simulink model "V2X_UDP_SCLX_Control_2019b"  (R2019b)
settings: Solver=FixedStepDiscrete  StartTime=0.0  StopTime=Inf  FixedStep=0.01  RelTol=1e-3
PostLoadFcn:
  | if any(exist('dsrtsu_mdlpostloadfcn', 'file') ~= 0), dsrtsu_mdlpostloadfcn('Execute', bdroot); end
InitFcn:
  | , if any(exist('rtifpga_mdlclblib', 'file') ~= 0), rtifpga_mdlclblib('Init', bdroot); end,
  | , if any(exist('dsmpb_private', 'file') ~= 0), dsmpb_private('dsmpb_mdlclblib', 'Init', bdroot); end,
values from neighbouring files (symbols this model uses):
  CtrlZone_Length = 250    [HDVPSG_DelayComp_NewRef_RealDrop_script_case1.m]
  High_TRFC = 1    [HDVPSG_DelayComp_NewRef_RealDrop_script_case1.m]
  PSG_AMAX = 3.2    [HDVPSG_DelayComp_NewRef_RealDrop_script_case1.m]
  PSG_AMIN = -6    [HDVPSG_DelayComp_NewRef_RealDrop_script_case1.m]
  PSG_first_v0 = 13    [HDVPSG_DelayComp_NewRef_RealDrop_script_case1.m]
  PSG_HighMu_D = 15    [HDVPSG_DelayComp_NewRef_RealDrop_script_case1.m]
  PSG_HighMu_I = 125    [HDVPSG_DelayComp_NewRef_RealDrop_script_case1.m]
  PSG_HighMu_P = 75    [HDVPSG_DelayComp_NewRef_RealDrop_script_case1.m]
  PSG_HighMu_TRFC = 0.8    [HDVPSG_DelayComp_NewRef_RealDrop_script_case1.m]
  PSG_LowMu_D = 12    [HDVPSG_DelayComp_NewRef_RealDrop_script_case1.m]
  PSG_LowMu_I = 64    [HDVPSG_DelayComp_NewRef_RealDrop_script_case1.m]
  PSG_LowMu_P = 48    [HDVPSG_DelayComp_NewRef_RealDrop_script_case1.m]
  PSG_LowMu_TRFC = 0.7    [HDVPSG_DelayComp_NewRef_RealDrop_script_case1.m]
  Q_Leader = 1    [HDVPSG_DelayComp_NewRef_RealDrop_script_case1.m]
  R_Leader = 20    [HDVPSG_DelayComp_NewRef_RealDrop_script_case1.m]
  T_ADE = 0.01    [HDVPSG_DelayComp_NewRef_RealDrop_script_case1.m]
  V_MAX = 40    [HDVPSG_DelayComp_NewRef_RealDrop_script_case1.m]
  V_MIN = 0    [HDVPSG_DelayComp_NewRef_RealDrop_script_case1.m]
undefined symbols (not defined in the file or in its folder): BETA_PSG_Leader, DiscIntNeverNeededParam, UT
libraries: simulink x4, dsmpblib x3
(part 1 of 3)
PreSaveFcn:
  | , if any(exist('dsmpb_private', 'file') ~= 0), dsmpb_private('dsmpb_mdlclblib', 'PreSave', bdroot); end,
CloseFcn:
  | , if any(exist('dsmpb_private', 'file') ~= 0), dsmpb_private('dsmpb_mdlclblib', 'Close', bdroot); end,
settings Model: DSRTSU_INTERNAL_RTIFPGA=200  DSRTSU_INTERNAL_RTISTBM_VER=22.2  DSMPB_ID_DATA={'1507',struct('BlockId','4137d8dd-4dad-4738-91c2-dd6ff22676c4','SignalIds',{{'2f3c0435-b5e6-43b5-a9a2-000eb5ecd229','997bbe15-e0e0-497e-95bc-98f0fbf39b57','0a3da5c5-423a-4b8d-b8d6-f3d0dcb59be2','87608d43-6927-4eb2-b378-ef61d2c19c9c','31e7d2b2-d685-4e77-a494-9395bd212b5d'}}),'1508',struct('BlockId','126ee60d-7173-4c59-ba7e-271ea2a4b692','SignalIds',{{'920c37f5-62e2-421b-87a3-b94423156c86','a9e93576-ca34-4bf6-b67a-2aec0185b5c4'}}),'1509',struct('BlockId','8da95892-a18c-4093-97c9-87f44c323683','SignalIds',{{'7a534e5d-6e34-444f-b618-91e9534136ef'}})}  Creator=znq  LastModifiedBy=Administrator
settings OptimizationCC: BlockReduction=off  ConditionallyExecuteInputs=off  OptimizeBlockIOStorage=off  BufferReuse=off
settings DebuggingCC: TasksWithSamePriorityMsg=none  UnconnectedInputMsg=none  UnconnectedOutputMsg=none  UnconnectedLineMsg=none  SFMachineParentedDataDiag=error
settings HardwareCC: ProdBitPerLong=64  ProdLargestAtomicInteger=Integer  ProdWordSize=32  ProdLongLongMode=on  ProdHWDeviceType=Custom Processor->Custom
settings ModelReferenceCC: EnableParallelModelReferenceBuilds=on
settings RTWCC: Description=dSPACE Target DSRT - Generates SIC files for import by ConfigurationDesk and VEOS. Provides code generation for Simulink models imported in ConfigurationDesk.  SystemTargetFile=dsrt.tlc  GenCodeOnly=on  MakeCommand=make_dsrt  TemplateMakefile=dsrt_default_tmf  RTWVerbose=off  TargetLang=C++
settings CodeAppCC: MaxIdLength=95
settings STFCustomTargetCC: TargetLangStandard=C++03 (ISO)  ParMdlRefBuildCompliant=on  SystemTargetFile=dsrt.tlc
settings GRTTargetCC: TargetLangStandard=C++03 (ISO)  CompOptLevelCompliant=off  ConcurrentExecutionCompliant=off  CombineOutputUpdateFcns=off  MatFileLogging=off  CPPClassGenCompliant=off  UseToolchainInfoCompliant=off

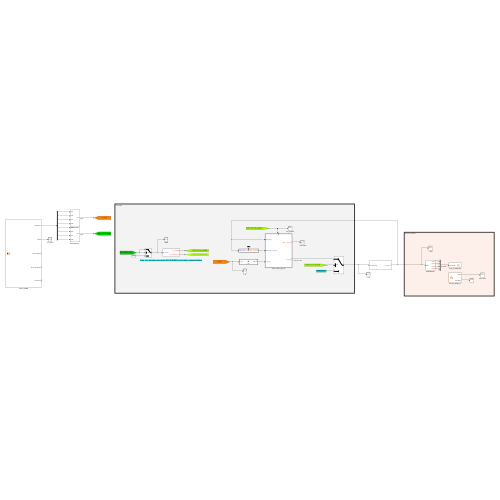
[thumbnail: Simulink's stored preview of the top-level diagram]
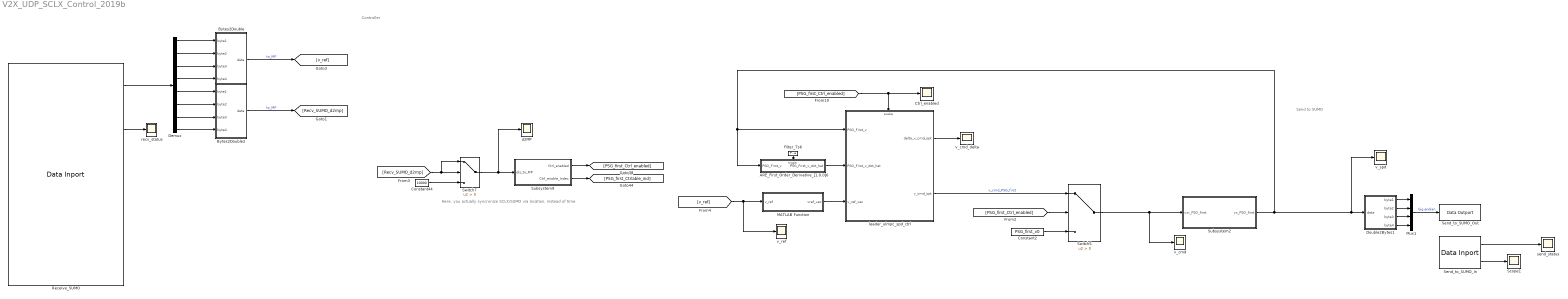
== system V2X_UDP_SCLX_Control_2019b ==
  note: Here, you actually syncronize SCLX/SUMO via location, instead of time
  note: Controller
  note: Send to SUMO
  ARE_First_Order_Derivative_[1,0,0]6 : Subsystem  TreatAsAtomicUnit=on
  Bytes2Double : Subsystem
  Bytes2Double2 : Subsystem
  Constant2 : Constant  Value=PSG_first_v0
  Constant44 : Constant  Value=10000
  Ctrl_enabled : Scope
  Demux : Demux  Outputs=8
  Double2Bytes1 : Subsystem
  Filter_Ts6 : DiscretePulseGenerator  PulseType=Time based  Period=T_ADE*2  PulseWidth=50
  MATLAB Function : MATLAB Function  TreatAsAtomicUnit=on
  Mux1 : Mux
  Receive_SUMO : dsmpblib/Data Inport  Priority=10000
      settings: SourceProductName=dSPACE Model Interface Package for Simulink (MIPS)
  Scope1 : Scope
  Send_to_SUMO_In : dsmpblib/Data Inport  Priority=10000
      settings: SourceProductName=dSPACE Model Interface Package for Simulink (MIPS)
  Send_to_SUMO_Out : dsmpblib/Data Outport  Priority=-10000
      settings: SourceProductName=dSPACE Model Interface Package for Simulink (MIPS)
  Subsystem2 : Subsystem
  Subsystem9 : Subsystem
  Switch5 : Switch  Criteria=u2 > Threshold
  Switch7 : Switch  Criteria=u2 > Threshold
  d2MP : Scope
  leader_ulmpc_spd_ctrl : Subsystem
  recv_status : Scope
  send_status : Scope
  v_cmd : Scope
  v_cmd_delta : Scope
  v_ref : Scope
  v_spd : Scope
  wires:
  Double2Bytes1/4(byte4) -> Mux1/4
  Double2Bytes1/3(byte3) -> Mux1/3
  Double2Bytes1/2(byte2) -> Mux1/2
  Double2Bytes1/1(byte1) -> Mux1/1
  Filter_Ts6/1 -> ARE_First_Order_Derivative_[1,0,0]6/Trigger
  Subsystem9/2(Ctrl_enable_Index) -> [PSG_first_Ctrlable_ind]
  Switch7/1 -> d2MP/1, Subsystem9/1(dis_to_MP)
  Constant44/1 -> Switch7/3
  [PSG_first_Ctrl_enabled] -> leader_ulmpc_spd_ctrl/Enable, Ctrl_enabled/1
  leader_ulmpc_spd_ctrl/2(v_cmd_opt) -> Switch5/1  "v_cmd_PSG_first"
  Subsystem9/1(Ctrl_enabled) -> [PSG_first_Ctrl_enabled]
  ARE_First_Order_Derivative_[1,0,0]6/1(PSG_First_v_dot_hat) -> leader_ulmpc_spd_ctrl/2(PSG_First_v_dot_hat)
  Constant2/1 -> Switch5/3
  [PSG_first_Ctrl_enabled] -> Switch5/2
  Switch5/1 -> v_cmd/1, Subsystem2/1(vxr_PSG_first)
  Mux1/1 -> Send_to_SUMO_Out/1  "big endian"
  leader_ulmpc_spd_ctrl/1(delta_v_cmd_opt) -> v_cmd_delta/1
  Subsystem2/1(vx_PSG_first) -> ARE_First_Order_Derivative_[1,0,0]6/1(PSG_First_v), leader_ulmpc_spd_ctrl/1(PSG_First_v), v_spd/1, Double2Bytes1/1(data)
  MATLAB Function/1(vref_vec) -> leader_ulmpc_spd_ctrl/3(v_ref_vec)
  [v_ref] -> v_ref/1, MATLAB Function/1(v_ref)
  Send_to_SUMO_In/1 -> send_status/1
  Send_to_SUMO_In/2 -> Scope1/1
  Receive_SUMO/1 -> Demux/1
  Receive_SUMO/2 -> recv_status/1
  Demux/1 -> Bytes2Double/1(byte1)
  Demux/2 -> Bytes2Double/2(byte2)
  Demux/3 -> Bytes2Double/3(byte3)
  Demux/4 -> Bytes2Double/4(byte4)
  Demux/5 -> Bytes2Double2/1(byte1)
  Demux/6 -> Bytes2Double2/2(byte2)
  Demux/7 -> Bytes2Double2/3(byte3)
  Demux/8 -> Bytes2Double2/4(byte4)
  Bytes2Double/1(data) -> [v_ref]  "to_MP"
  Bytes2Double2/1(data) -> [Recv_SUMO_d2mp]  "to_MP"
  [Recv_SUMO_d2mp] -> Switch7/1, Switch7/2

== system V2X_UDP_SCLX_Control_2019b/ARE_First_Order_Derivative_[1,0,0]6 ==
  PSG_First_v : Inport
  Trigger : TriggerPort  TriggerType=either  VariantControl=Variant  ZeroCross=off  PortDimensions=1
  Constant : Constant  Value=T_ADE
  Constant1 : Constant  Value=PSG_first_v0
  MATLAB Function : MATLAB Function  TreatAsAtomicUnit=on
  PSG_First_v_dot_hat : Outport  VectorParamsAs1DForOutWhenUnconnected=off
  wires:
  Constant1/1 -> MATLAB Function/3(u_init)
  PSG_First_v/1 -> MATLAB Function/1(U)
  MATLAB Function/1(Dot_U) -> PSG_First_v_dot_hat/1
  Constant/1 -> MATLAB Function/2(Ts)

== system V2X_UDP_SCLX_Control_2019b/Bytes2Double ==
  byte1 : Inport
  byte2 : Inport  Port=2
  byte3 : Inport  Port=3
  byte4 : Inport  Port=4
  Data Type Conversion2 : DataTypeConversion
  MATLAB Function2 : MATLAB Function  TreatAsAtomicUnit=on
  data : Outport
  wires:
  byte1/1 -> MATLAB Function2/1(byte1)
  byte3/1 -> MATLAB Function2/3(byte3)
  MATLAB Function2/1(float32) -> Data Type Conversion2/1
  byte4/1 -> MATLAB Function2/4(byte4)
  Data Type Conversion2/1 -> data/1
  byte2/1 -> MATLAB Function2/2(byte2)

== system V2X_UDP_SCLX_Control_2019b/Bytes2Double2 ==
  byte1 : Inport
  byte2 : Inport  Port=2
  byte3 : Inport  Port=3
  byte4 : Inport  Port=4
  Data Type Conversion2 : DataTypeConversion
  MATLAB Function2 : MATLAB Function  TreatAsAtomicUnit=on
  data : Outport
  wires:
  byte2/1 -> MATLAB Function2/2(byte2)
  Data Type Conversion2/1 -> data/1
  byte4/1 -> MATLAB Function2/4(byte4)
  MATLAB Function2/1(float32) -> Data Type Conversion2/1
  byte3/1 -> MATLAB Function2/3(byte3)
  byte1/1 -> MATLAB Function2/1(byte1)

== system V2X_UDP_SCLX_Control_2019b/Double2Bytes1 ==
  data : Inport
  MATLAB Function3 : MATLAB Function  TreatAsAtomicUnit=on
  Saturation : Saturate  UpperLimit=1e6  LowerLimit=-1e6
  byte1 : Outport
  byte2 : Outport  Port=2
  byte3 : Outport  Port=3
  byte4 : Outport  Port=4
  wires:
  Saturation/1 -> MATLAB Function3/1(defloatMe)
  MATLAB Function3/4(byte4) -> byte4/1
  MATLAB Function3/1(byte1) -> byte1/1
  MATLAB Function3/2(byte2) -> byte2/1
  data/1 -> Saturation/1
  MATLAB Function3/3(byte3) -> byte3/1

== system V2X_UDP_SCLX_Control_2019b/Subsystem2 ==
  vxr_PSG_first : Inport
  Constant56 : Constant  Value=PSG_first_v0
  PSG_first : Subsystem
  Subsystem4 : Subsystem
  Subsystem5 : Subsystem
  Subsystem6 : Subsystem
  Subsystem7 : Subsystem
  Terminator : Terminator
  vx_PSG_first : Outport
  wires:
  vxr_PSG_first/1 -> PSG_first/1(vxr)
  Constant56/1 -> PSG_first/6(v_ini)
  Subsystem4/1(PSG_P) -> PSG_first/2(PID_P)
  Subsystem5/1(PSG_I) -> PSG_first/3(PID_I)
  Subsystem6/1(PSG_D) -> PSG_first/4(PID_D)
  Subsystem7/1(PSG_Mu) -> PSG_first/5(TRFC)
  PSG_first/1(vx) -> vx_PSG_first/1
  PSG_first/2(ax_) -> Terminator/1

== system V2X_UDP_SCLX_Control_2019b/Subsystem9 ==
  dis_to_MP : Inport
  Add5 : Sum
  Compare To Constant1 : simulink/Logic and Bit Operations/Compare To Constant  relop=<=  const=CtrlZone_Length  OutDataTypeStr=boolean
  Compare To Constant2 : simulink/Logic and Bit Operations/Compare To Constant  relop=>  const=0  OutDataTypeStr=boolean
  Data Type Conversion : DataTypeConversion
  Delay : Delay  DelayLength=1
  Ctrl_enabled : Outport
  Ctrl_enable_Index : Outport  Port=2
  wires:
  Data Type Conversion/1 -> Add5/1
  Delay/1 -> Ctrl_enable_Index/1, Add5/2, Compare To Constant2/1
  Add5/1 -> Delay/1
  Compare To Constant2/1 -> Ctrl_enabled/1
  Compare To Constant1/1 -> Data Type Conversion/1
  dis_to_MP/1 -> Compare To Constant1/1

== system V2X_UDP_SCLX_Control_2019b/leader_ulmpc_spd_ctrl ==
  note: CVXGEN only support C compiler. So, this is another reason why you cannot build CVXGEN and SUMO (C++11) code together into SCLX
  note: After test the CVXGEN in a complete Simulink model, you need to separate the CVXGEN file into a Ctrl.slx file to be built into SCLX.
      |
      | Please first delete the generated CVXGEN file from the last local compilation.
      | After you analyze the Ctrl.slx, you will find the CVXGEN related wrapper, etc will automatically appear. Then, make sure the Code Gen setup in Simulink is set to C, instead of C++. Then, you can let CfgDesk to build.
  PSG_First_v : Inport
  PSG_First_v_dot_hat : Inport  Port=2
  v_ref_vec : Inport  Port=3
  Enable : EnablePort
  Constant42 : Constant  Value=Q_Leader
  Constant43 : Constant  Value=R_Leader
  Constant54 : Constant  Value=PSG_AMAX*T_ADE
  Constant55 : Constant  Value=PSG_AMIN*T_ADE
  Constant57 : Constant  Value=V_MAX
  Constant58 : Constant  Value=V_MIN
  Constant59 : Constant  Value=T_ADE
  Constant61 : Constant  Value=BETA_PSG_Leader
  Memory2 : Memory  InitialCondition=PSG_first_v0
  Rate Transition{6,48..50,68,70..80} (16 alike) : RateTransition
  S-Function Builder : S-Function  FunctionName=ULMPC_Spd_Ctrl  SFunctionModules=ULMPC_Spd_Ctrl_wrapper solver util matrix_support ldl  SFunctionDeploymentMode=off  EnableBusSupport=off  mask(S-Function Builder){}
      mask help: Simulink:masks:SFunctionBuilder_MD
      mask init:
      | val = [[.9  0.75 0.75 1 1 .9 .9 1]',[1 1 0.75 0.75 .9 .9 1 .9]'];try , sys = get_param(gcb,'SfunBuilderFcnName');if isempty(sys), sys = get_param(gcb,'FunctionName'); end,catch, sys = get_param(gcb,'FunctionName'); end
      settings: CopyFcn=set_param(gcbh,'LinkStatus','none')  OpenFcn=sfunctionwizard(gcbh)
      mask Display:
      | plot(val(:,1),val(:,2))
      | disp(sys)
      | port_label('input',1,'vmax')
      | port_label('input',2,'vmin')
      | port_label('input',3,'deltav_max')
      | port_label('input',4,'deltav_min')
      | port_label('input',5,'vcmd_max')
      | port_label('input',6,'vcmd_min')
      | port_label('input',7,'delta_vcmd_max')
      | port_label('input',8,'delta_vcmd_min')
      | port_label('input',9,'A')
      | port_label('input',10,'B')
      | port_label('input',11,'d_k')
      | port_label('input',12,'Q')
      | port_label('input',13,'R')
      | port_label('input',14,'v_ref')
      | port_label('input',15,'v_cmd_last')
      | port_label('input',16,'x_0')
      | port_label('output',1,'delta_v_cmd_opt')
      | port_label('output',2,'v_cmd_opt')
  Scope : Scope
  Sys_Leader : MATLAB Function  TreatAsAtomicUnit=on
  delta_v_cmd_opt : Outport
  v_cmd_opt : Outport  Port=2
  wires:
  S-Function Builder/2 -> v_cmd_opt/1, Memory2/1  "v_cmd_opt"
  Sys_Leader/3(dk) -> Rate Transition48/1
  Rate Transition49/1 -> S-Function Builder/1
  Rate Transition50/1 -> S-Function Builder/2
  Constant61/1 -> Sys_Leader/2(beta)
  Sys_Leader/2(B) -> Rate Transition72/1
  Rate Transition77/1 -> S-Function Builder/7
  Constant59/1 -> Sys_Leader/1(Ts)
  Rate Transition75/1 -> S-Function Builder/13
  Constant55/1 -> Rate Transition70/1, Rate Transition78/1
  Constant54/1 -> Rate Transition68/1, Rate Transition77/1
  Rate Transition48/1 -> S-Function Builder/11
  Rate Transition72/1 -> S-Function Builder/10
  Rate Transition68/1 -> S-Function Builder/3
  Rate Transition70/1 -> S-Function Builder/4
  Constant58/1 -> Rate Transition50/1, Rate Transition76/1
  Rate Transition74/1 -> S-Function Builder/12
  Rate Transition76/1 -> S-Function Builder/6
  Constant57/1 -> Rate Transition49/1, Rate Transition73/1
  Constant42/1 -> Rate Transition74/1
  Rate Transition6/1 -> S-Function Builder/16
  Sys_Leader/1(A) -> Rate Transition71/1
  S-Function Builder/1 -> Scope/1, delta_v_cmd_opt/1
  Rate Transition71/1 -> S-Function Builder/9
  Rate Transition73/1 -> S-Function Builder/5
  Memory2/1 -> Rate Transition80/1
  Rate Transition80/1 -> S-Function Builder/15
  Rate Transition78/1 -> S-Function Builder/8
  Rate Transition79/1 -> S-Function Builder/14  "21"
  PSG_First_v/1 -> Rate Transition6/1
  Constant43/1 -> Rate Transition75/1
  PSG_First_v_dot_hat/1 -> Sys_Leader/3(v_dot_hat)
  v_ref_vec/1 -> Rate Transition79/1

== system V2X_UDP_SCLX_Control_2019b/Subsystem2/PSG_first ==
  note: [v: 0--13--20]
      | High Frict PSG: P=75, I=125, D=15, TRFC=0.8 -->   -7.2<a<4.4
      | Low Frict  PSG: P=48, I=64,   D=12, TRFC=0.7 -->   -6.0<a<3.2
      |
      | High Frict HDV: P=27, I=27, D=9, TRFC=0.7 -->  -4.3<a<2.2
      | Low Frict  HDV: P=12, I=8,   D=6, TRFC=0.6 -->  -2.5<a<1.3
      |
      | ULMPC treat sudden drop of TRFC!
  vxr : Inport
  PID_P : Inport  Port=2
  PID_I : Inport  Port=3
  PID_D : Inport  Port=4
  TRFC : Inport  Port=5
  v_ini : Inport  Port=6
  Body Fixed Vehicle Dynamics : Subsystem
  Constant{1..5} (5 alike) : Constant  Value=0
  Cruise Speed Control : Subsystem
  Gain{,1..3} (4 alike) : Gain  Gain=UT.Rw
  Global Coordinates : Subsystem
  Scope : Scope
  Scope1 : Scope
  Scope3 : Scope
  Terminator : Terminator
  Vx : Scope
  X : Scope
  Y : Scope
  ax : Scope
  ay : Scope
  deg/rad : Gain  Gain=pi/180
  deg/rad1 : Gain  Gain=pi/180
  left/right wheel steer : Subsystem
  omegafl : Scope
  omegafr : Scope
  omegarl : Scope
  omegarr : Scope
  vy : Scope
  yaw : Scope
  yaw_rate : Scope
  vx : Outport
  ax_ : Outport  Port=2
  wires:
  Constant5/1 -> Body Fixed Vehicle Dynamics/9(vy_ini)
  Constant2/1 -> Body Fixed Vehicle Dynamics/8(yaw_ini)
  v_ini/1 -> Body Fixed Vehicle Dynamics/7(V_ini)
  TRFC/1 -> Body Fixed Vehicle Dynamics/6(TRFC)
  PID_D/1 -> Cruise Speed Control/5(PID_D)
  PID_I/1 -> Cruise Speed Control/4(PID_I)
  PID_P/1 -> Cruise Speed Control/3(PID_P)
  Global Coordinates/1(X) -> X/1
  Body Fixed Vehicle Dynamics/6(Vx) -> vx/1, Cruise Speed Control/1(Vx), Vx/1, Global Coordinates/2(Vx)
  Body Fixed Vehicle Dynamics/3(omegarl) -> Gain2/1
  Body Fixed Vehicle Dynamics/4(omegarr) -> Gain3/1
  Body Fixed Vehicle Dynamics/1(omegafl) -> Gain/1
  Body Fixed Vehicle Dynamics/10(Vy) -> vy/1, Global Coordinates/3(Vy)
  Cruise Speed Control/1(Throttle) -> Scope1/1, Body Fixed Vehicle Dynamics/1(Tdf)
  Gain2/1 -> omegarl/1
  Gain/1 -> omegafl/1
  Body Fixed Vehicle Dynamics/7("Yaw Rate ") -> yaw_rate/1
  Body Fixed Vehicle Dynamics/12(Sideslip Angle Alpha) -> Scope/1
  vxr/1 -> Cruise Speed Control/2(Vxr)
  Gain1/1 -> omegafr/1
  Body Fixed Vehicle Dynamics/9(ay) -> ay/1
  Body Fixed Vehicle Dynamics/11(Beta) -> Terminator/1
  deg/rad/1 -> Body Fixed Vehicle Dynamics/4(deltaFL)
  Constant1/1 -> left/right wheel steer/1(steering wheel angle deg)
  Body Fixed Vehicle Dynamics/2(omegafr) -> Gain1/1
  Global Coordinates/2(Y) -> Y/1
  Gain3/1 -> omegarr/1
  deg/rad1/1 -> Body Fixed Vehicle Dynamics/3(deltaFR), Scope3/1
  left/right wheel steer/1(Right wheel steer ground (deg)) -> deg/rad1/1
  left/right wheel steer/2(Left wheel steer ground (deg)) -> deg/rad/1
  Body Fixed Vehicle Dynamics/8(Yaw Angle) -> Global Coordinates/1(Heading Angle), yaw/1
  Body Fixed Vehicle Dynamics/5(ax) -> ax/1, ax_/1
  Constant3/1 -> Body Fixed Vehicle Dynamics/5(slope)
  Constant4/1 -> Body Fixed Vehicle Dynamics/2(Brake)

== system V2X_UDP_SCLX_Control_2019b/Subsystem2/Subsystem4 ==
  Constant56 : Constant  Value=High_TRFC
  Constant57 : Constant  Value=PSG_HighMu_P
  Constant58 : Constant  Value=PSG_LowMu_P
  Switch : Switch  Criteria=u2 > Threshold
  PSG_P : Outport
  wires:
  Switch/1 -> PSG_P/1
  Constant58/1 -> Switch/3
  Constant57/1 -> Switch/1
  Constant56/1 -> Switch/2

== system V2X_UDP_SCLX_Control_2019b/Subsystem2/Subsystem5 ==
  Constant56 : Constant  Value=High_TRFC
  Constant57 : Constant  Value=PSG_HighMu_I
  Constant58 : Constant  Value=PSG_LowMu_I
  Switch : Switch  Criteria=u2 > Threshold
  PSG_I : Outport
  wires:
  Constant56/1 -> Switch/2
  Constant57/1 -> Switch/1
  Constant58/1 -> Switch/3
  Switch/1 -> PSG_I/1

== system V2X_UDP_SCLX_Control_2019b/Subsystem2/Subsystem6 ==
  Constant56 : Constant  Value=High_TRFC
  Constant57 : Constant  Value=PSG_HighMu_D
  Constant58 : Constant  Value=PSG_LowMu_D
  Switch : Switch  Criteria=u2 > Threshold
  PSG_D : Outport
  wires:
  Switch/1 -> PSG_D/1
  Constant58/1 -> Switch/3
  Constant57/1 -> Switch/1
  Constant56/1 -> Switch/2

== system V2X_UDP_SCLX_Control_2019b/Subsystem2/Subsystem7 ==
  Constant1 : Constant  Value=PSG_LowMu_TRFC
  Constant2 : Constant  Value=High_TRFC
  Constant57 : Constant  Value=PSG_HighMu_TRFC
  Switch : Switch  Criteria=u2 > Threshold
  PSG_Mu : Outport
  wires:
  Constant57/1 -> Switch/1
  Constant1/1 -> Switch/3
  Switch/1 -> PSG_Mu/1
  Constant2/1 -> Switch/2

== system V2X_UDP_SCLX_Control_2019b/Subsystem2/PSG_first/Body Fixed Vehicle Dynamics ==
  Tdf : Inport
  Brake : Inport  Port=2
  deltaFR : Inport  Port=3
  deltaFL : Inport  Port=4
  slope : Inport  Port=5
  TRFC : Inport  Port=6
  V_ini : Inport  Port=7
  yaw_ini : Inport  Port=8
  vy_ini : Inport  Port=9
  8dof_vehicle : Subsystem
  Brakes : Subsystem
  Bus Creator{,2..4} (4 alike) : BusCreator  Inputs=4
  Bus Creator1 : BusCreator  Inputs=8
  Bus Creator5 : BusCreator  Inputs=3
  Bus Selector : BusSelector  OutputSignals=signal1,signal2,signal3,signal4
  Constant : Constant  Value=0
  Constant1 : Constant  Value=0
  Driving Resistance Subsystem : Subsystem
  Fz : Subsystem
  Magic Formula Tire Model1 : Subsystem
  "Tire Longitudinal Center Speed " : Subsystem
  Tire Sideslip Angle : Subsystem
  To Workspace : ToWorkspace  VariableName=PSG1_FxFL  SaveFormat=Timeseries  SampleTime=-1
  To Workspace1 : ToWorkspace  VariableName=PSG1_FxRL  SaveFormat=Timeseries  SampleTime=-1
  To Workspace2 : ToWorkspace  VariableName=PSG1_FxFR  SaveFormat=Timeseries  SampleTime=-1
  To Workspace3 : ToWorkspace  VariableName=PSG1_FxRR  SaveFormat=Timeseries  SampleTime=-1
  Unit Delay : UnitDelay  SampleTime=UT.Ts_Veh  HasFrameUpgradeWarning=on
  Unit Delay1 : UnitDelay  SampleTime=UT.Ts_Veh  HasFrameUpgradeWarning=on
  deltaFL1 : InportShadow  Port=4
  deltaFL2 : InportShadow  Port=4
  deltaFR1 : InportShadow  Port=3
  deltaFR2 : InportShadow  Port=3
  lamda slip ratio : Subsystem
  omegafl : Outport  VectorParamsAs1DForOutWhenUnconnected=off
  omegafr : Outport  Port=2  VectorParamsAs1DForOutWhenUnconnected=off
  omegarl : Outport  Port=3  VectorParamsAs1DForOutWhenUnconnected=off
  omegarr : Outport  Port=4  VectorParamsAs1DForOutWhenUnconnected=off
  ax : Outport  Port=5  VectorParamsAs1DForOutWhenUnconnected=off
  Vx : Outport  Port=6  VectorParamsAs1DForOutWhenUnconnected=off
  "Yaw Rate " : Outport  Port=7  VectorParamsAs1DForOutWhenUnconnected=off
  Yaw Angle : Outport  Port=8  VectorParamsAs1DForOutWhenUnconnected=off
  ay : Outport  Port=9  VectorParamsAs1DForOutWhenUnconnected=off
  Vy : Outport  Port=10  VectorParamsAs1DForOutWhenUnconnected=off
  Beta : Outport  Port=11  VectorParamsAs1DForOutWhenUnconnected=off
  Sideslip Angle Alpha : Outport  Port=12  VectorParamsAs1DForOutWhenUnconnected=off
  wires:
  8dof_vehicle/15(Roll Rate) -> Fz/9(roll rate)
  vy_ini/1 -> 8dof_vehicle/14(vy_ini)
  yaw_ini/1 -> 8dof_vehicle/13(yaw_ini)
  V_ini/1 -> 8dof_vehicle/12(V_ini)
  TRFC/1 -> Magic Formula Tire Model1/2(TRFC)
  Bus Creator/1 -> Bus Selector/1
  Tdf/1 -> 8dof_vehicle/1(Tdf)
  8dof_vehicle/1(omegafl) -> omegafl/1, lamda slip ratio/1(omegafl)
  8dof_vehicle/2(omegafr) -> omegafr/1, lamda slip ratio/2(omegafr)
  8dof_vehicle/3(omegarl) -> omegarl/1, lamda slip ratio/3(omegarl)
  8dof_vehicle/4(omegarr) -> omegarr/1, lamda slip ratio/4(omegarr)
  8dof_vehicle/8(Yaw angle) -> Yaw Angle/1
  Bus Creator1/1 -> 8dof_vehicle/6(In7)
  8dof_vehicle/10(Vy) -> Vy/1, Tire Sideslip Angle/1(Vy), "Tire Longitudinal Center Speed "/2(Vy)
  Magic Formula Tire Model1/2(Fy_FL) -> Bus Creator1/2
  Magic Formula Tire Model1/1(Fx_FL) -> To Workspace/1, Bus Creator1/1
  Fz/4(Fzrr) -> Bus Creator3/4
  Fz/3(Fzrl) -> Bus Creator3/3
  Fz/2(Fzfr) -> Bus Creator3/2
  Fz/1(Fzfl) -> Bus Creator3/1
  Bus Creator2/1 -> Bus Creator5/1, Brakes/1(lambda)  "lamda"
  Bus Creator4/1 -> Bus Creator5/3  "alpha"
  Bus Creator5/1 -> Magic Formula Tire Model1/1(VehState)
  Tire Sideslip Angle/4(alpha_rr: rad) -> Bus Creator4/4
  Tire Sideslip Angle/3(alpha_rl: rad) -> Bus Creator4/3
  Tire Sideslip Angle/1(alpha_fl: rad) -> Bus Creator4/1, Sideslip Angle Alpha/1
  Tire Sideslip Angle/2(alpha_fr: rad) -> Bus Creator4/2
  "Tire Longitudinal Center Speed "/4(Vwrr) -> Bus Creator/4
  "Tire Longitudinal Center Speed "/2(Vwfr) -> Bus Creator/2
  "Tire Longitudinal Center Speed "/1(Vwfl) -> Bus Creator/1
  "Tire Longitudinal Center Speed "/3(Vwrl) -> Bus Creator/3
  Bus Selector/1 -> lamda slip ratio/5(Vwfl)  "<signal1>"
  Bus Selector/2 -> lamda slip ratio/6(Vwfr)  "<signal2>"
  Bus Selector/3 -> lamda slip ratio/7(Vwrl)  "<signal3>"
  Bus Selector/4 -> lamda slip ratio/8(Vwrr)  "<signal4>"
  Driving Resistance Subsystem/2(Fr) -> 8dof_vehicle/8(Fr)
  deltaFL/1 -> lamda slip ratio/9(deltaFL)  "deltaw"
  deltaFL1/1 -> Tire Sideslip Angle/4(deltaFL)  "deltaw"
  8dof_vehicle/9(ay) -> ay/1, Unit Delay1/1
  8dof_vehicle/11("Veh Sideslip, Beta") -> "Tire Longitudinal Center Speed "/4(VehSideSlip Beta), Beta/1, Tire Sideslip Angle/6(Beta)
  8dof_vehicle/6(Vx) -> Vx/1, Driving Resistance Subsystem/1(Vx), Tire Sideslip Angle/3(Vx), "Tire Longitudinal Center Speed "/1(Vx)
  8dof_vehicle/7(Yaw Rate) -> "Yaw Rate "/1, Tire Sideslip Angle/2(Yaw Rate), "Tire Longitudinal Center Speed "/3(YawRate)
  slope/1 -> 8dof_vehicle/9(slope)
  Constant1/1 -> Fz/6(bank angle)
  Driving Resistance Subsystem/1(Fax) -> Fz/1(Fa), 8dof_vehicle/7(Fax)
  Constant/1 -> Fz/3(slope)
  8dof_vehicle/5(ax) -> ax/1, Unit Delay/1
  deltaFL2/1 -> 8dof_vehicle/10(deltaFL)  "deltaw"
  Magic Formula Tire Model1/5(Fx_RL) -> To Workspace1/1, Bus Creator1/5
  Magic Formula Tire Model1/7(Fx_RR) -> To Workspace3/1, Bus Creator1/7
  Magic Formula Tire Model1/8(Fy_RR) -> Bus Creator1/8
  Magic Formula Tire Model1/6(Fy_RL) -> Bus Creator1/6
  Magic Formula Tire Model1/3(Fx_FR) -> To Workspace2/1, Bus Creator1/3
  Magic Formula Tire Model1/4(Fy_FR) -> Bus Creator1/4
  Unit Delay1/1 -> Fz/5(ay)
  Unit Delay/1 -> Fz/2(ax)
  lamda slip ratio/1(lamdafl) -> Bus Creator2/1
  lamda slip ratio/2(lamdafr) -> Bus Creator2/2
  lamda slip ratio/3(lamdarl) -> Bus Creator2/3
  lamda slip ratio/4(lamdarr) -> Bus Creator2/4
  deltaFR/1 -> lamda slip ratio/10(deltaFR)
  deltaFR1/1 -> Tire Sideslip Angle/5(deltaFR1)
  deltaFR2/1 -> 8dof_vehicle/11(deltaRL)
  Bus Creator3/1 -> Bus Creator5/2
  8dof_vehicle/13(Pitch_rate) -> Fz/8(pitch rate)
  8dof_vehicle/12(Pitch) -> Fz/4(pitch angle)
  8dof_vehicle/14("Roll ") -> Fz/7(roll angle)
  Brake/1 -> Brakes/2(brake postion)
  Brakes/1(Tbfl) -> 8dof_vehicle/2(Tbfl)
  Brakes/2(Tbfr) -> 8dof_vehicle/3(Tbfr)
  Brakes/3(Tbrl) -> 8dof_vehicle/4(Tbrl)
  Brakes/4(Tbrr) -> 8dof_vehicle/5(Tbrr)

== system V2X_UDP_SCLX_Control_2019b/Subsystem2/PSG_first/Cruise Speed Control ==
  Vx : Inport
  Vxr : Inport  Port=2
  PID_P : Inport  Port=3
  PID_I : Inport  Port=4
  PID_D : Inport  Port=5
  Constant : Constant  Value=100
  Gain : Gain  Gain=2
  PID Controller : simulink/Continuous/PID Controller  Controller=PID  Form=Parallel  TimeDomain=Discrete-time  SampleTime=UT.Ts_Veh  IntegratorMethod=Forward Euler  FilterMethod=Forward Euler  ControllerParametersSource=external  P=UT.PID_P_PSG  I=UT.PID_I_PSG  D=UT.PID_D_PSG  N=100  UseFilter=on  TunerSelectOption=Transfer Function Based (PID Tuner App)  InitialConditionSource=internal  InitialConditionForIntegrator=0  InitialConditionForFilter=0  DifferentiatorICPrevScaledInput=0  ExternalReset=none  TrackingMode=off  Kt=1  LimitOutput=off  UpperSaturationLimit=inf  LowerSaturationLimit=-inf  LinearizeAsGain=on  AntiWindupMode=none  Kb=1  POutMin=[]  POutMax=[]  IOutMin=[]  IOutMax=[]  DOutMin=[]  DOutMax=[]  NOutMin=[]  NOutMax=[]  SumOutMin=[]  SumOutMax=[]  SaturationOutMin=[]  SaturationOutMax=[]  PParamMin=[]  PParamMax=[]  IParamMin=[]  IParamMax=[]  DParamMin=[]  DParamMax=[]  NParamMin=[]  NParamMax=[]  KbParamMin=[]  KbParamMax=[]  KtParamMin=[]  KtParamMax=[]  KbOutMin=[]  KbOutMax=[]  KtOutMin=[]  KtOutMax=[]  IntegratorOutMin=[]  IntegratorOutMax=[]  FilterOutMin=[]  FilterOutMax=[]  SumI1OutMin=[]  SumI1OutMax=[]  SumI2OutMin=[]  SumI2OutMax=[]  SumI3OutMin=[]  SumI3OutMax=[]  SumI4OutMin=[]  SumI4OutMax=[]  SumDOutMin=[]  SumDOutMax=[]  DifferentiatorOutMin=[]  DifferentiatorOutMax=[]  FilterDiffOutCoefMin=[]  FilterDiffOutCoefMax=[]  ReciprocalOutMin=[]  ReciprocalOutMax=[]  SumDenOutMin=[]  SumDenOutMax=[]  SumNumOutMin=[]  SumNumOutMax=[]  DivideOutMin=[]  DivideOutMax=[]  IntegratorContinuousStateAttributes=''  IntegratorStateMustResolveToSignalObject=off  IntegratorRTWStateStorageClass=Auto  FilterContinuousStateAttributes=''  FilterStateMustResolveToSignalObject=off  FilterRTWStateStorageClass=Auto  ParallelPVariant=ExternalParameters  IdealPVariant=Disabled  IVariant=ExternalParameters  DVariant=ExternalParameters  IntegratorVariant=Discrete  SatVariant=Disabled  AWVariant=Passthrough  PCopyVariant=Disabled  TRVariant=Disabled  FdbkBlocksVariant=Forward  IdealPFdbkVariant=Disabled  SatFdbkVariant=Disabled  DerivativeFilterVariant=ForwardEulerFilter  NVariant=ExternalParameters  NCopyVariant=Disabled  FilterICVariant=InternalICsFilter  IntegratorICVariant=InternalICs  ExternalResetVariant=Disabled  TRSumVariant=Passthrough  SumFdbkVariant=Disabled  SumVariant=Sum_PID
  Subtract : Sum  Inputs=-+
  Throttle : Outport  VectorParamsAs1DForOutWhenUnconnected=off
  wires:
  PID_D/1 -> PID Controller/4
  PID_I/1 -> PID Controller/3
  PID_P/1 -> PID Controller/2
  Constant/1 -> PID Controller/5
  PID Controller/1 -> Gain/1
  Subtract/1 -> PID Controller/1
  Gain/1 -> Throttle/1
  Vxr/1 -> Subtract/2
  Vx/1 -> Subtract/1

== system V2X_UDP_SCLX_Control_2019b/Subsystem2/PSG_first/Global Coordinates ==
  Heading Angle : Inport
  Vx : Inport  Port=2
  Vy : Inport  Port=3
  Add : Sum
  Discrete-Time Integrator : DiscreteIntegrator  SampleTime=UT.Ts_Veh  ICPrevOutput=DiscIntNeverNeededParam  ICPrevScaledInput=DiscIntNeverNeededParam
  Discrete-Time Integrator1 : DiscreteIntegrator  SampleTime=UT.Ts_Veh  ICPrevOutput=DiscIntNeverNeededParam  ICPrevScaledInput=DiscIntNeverNeededParam
  Math Function : Math  Operator=square  SignedPower=on  SaturateOnIntegerOverflow=on
  Math Function1 : Math  Operator=square  SignedPower=on  SaturateOnIntegerOverflow=on
  Product{,1..3} (4 alike) : Product
  Sign : Signum
  Sign1 : Signum
  Sqrt : Sqrt  Operator=signedSqrt  SaturateOnIntegerOverflow=on
  Trigonometric Function : Trigonometry
  Trigonometric Function1 : Trigonometry  Operator=cos
  X : Outport  VectorParamsAs1DForOutWhenUnconnected=off
  Y : Outport  Port=2  VectorParamsAs1DForOutWhenUnconnected=off
  wires:
  Vx/1 -> Math Function/1, Sign/1
  Vy/1 -> Math Function1/1, Sign1/1
  Add/1 -> Sqrt/1
  Heading Angle/1 -> Trigonometric Function1/1, Trigonometric Function/1
  Sqrt/1 -> Product1/2, Product/2
  Trigonometric Function1/1 -> Product/1
  Trigonometric Function/1 -> Product1/1
  Product/1 -> Discrete-Time Integrator1/1
  Product1/1 -> Discrete-Time Integrator/1
  Discrete-Time Integrator1/1 -> X/1
  Discrete-Time Integrator/1 -> Y/1
  Math Function/1 -> Product2/1
  Sign/1 -> Product2/2
  Product2/1 -> Add/1
  Math Function1/1 -> Product3/1
  Sign1/1 -> Product3/2
  Product3/1 -> Add/2

== system V2X_UDP_SCLX_Control_2019b/Subsystem2/PSG_first/left//right wheel steer ==
  steering wheel angle deg : Inport
  Deadband Deg : DeadZone  LowerValue=-2  UpperValue=2  SaturateOnIntegerOverflow=on
  Gain : Gain  Gain=0.9
  Gain1 : Gain  Gain=0.9
  Left wheel rack displacement to ground steering angle1 : Lookup_n-D  NumberOfTableDimensions=1  BreakpointsForDimension1=|  Table=|  RndMeth=Simplest  InputSameDT=on
      | [-83.31
      | -80.10576923
      | -77.13888889
      | -74.38392857
      | -71.81896552
      | -69.425
      | -67.18548387
      | -65.0859375
      | -63.11363636
      | -61.25735294
      | -59.50714286
      | -57.85416667
      | -56.29054054
      | -54.80921053
      | -53.40384615
      | -52.06875
      | -50.79878049
      | -49.58928571
      | -48.43604651
      | -47.33522727
      | -46.28333333
      | -45.27717391
      | -44.31382979
      | -43.390625
      | -42.50510204
      | -41.655
      | 0
      | 41.655
      | 42.50510204
      | 43.390625
      | 44.31382979
      | 45.27717391
      | 46.28333333
      | 47.33522727
      | 48.43604651
      | 49.58928571
      | 50.79878049
      | 52.06875
      | 53.40384615
      | 54.80921053
      | 56.29054054
      | 57.85416667
      | 59.50714286
      | 61.25735294
      | 63.11363636
      | 65.0859375
      | 67.18548387
      | 69.425
      | 71.81896552
      | 74.38392857
      | 77.13888889
      | 80.10576923
      | 83.31
      | ]
      | [-39.37720355
      | -37.63494871
      | -36.07707064
      | -34.67025898
      | -33.38971041
      | -32.21639355
      | -31.13534711
      | -30.13457154
      | -29.20427963
      | -28.33637359
      | -27.52407048
      | -26.76162747
      | -26.04413644
      | -25.36736764
      | -24.72764882
      | -24.12177053
      | -23.54691095
      | -23.00057556
      | -22.48054833
      | -21.98485165
      | -21.51171342
      | -21.05953958
      | -20.62689117
      | -20.21246499
      | -19.81507719
      | -19.43364926
      | 0
      | 23.71741561
      | 24.27669186
      | 24.86323253
      | 25.47909206
      | 26.1265372
      | 26.80807528
      | 27.52648702
      | 28.28486498
      | 29.08665866
      | 29.93572777
      | 30.83640531
      | 31.7935729
      | 32.81275112
      | 33.9002085
      | 35.06309421
      | 36.30960068
      | 37.64916478
      | 39.09271935
      | 40.65301137
      | 42.34501024
      | 44.1864403
      | 46.19848973
      | 48.40677775
      | 50.84271532
      | 53.54549481
      | 56.56514507
      | ]
  Right wheel rack displacement to ground steering angle : Lookup_n-D  NumberOfTableDimensions=1  BreakpointsForDimension1=|  Table=|  RndMeth=Simplest  InputSameDT=on
      | [-83.31
      | -80.10576923
      | -77.13888889
      | -74.38392857
      | -71.81896552
      | -69.425
      | -67.18548387
      | -65.0859375
      | -63.11363636
      | -61.25735294
      | -59.50714286
      | -57.85416667
      | -56.29054054
      | -54.80921053
      | -53.40384615
      | -52.06875
      | -50.79878049
      | -49.58928571
      | -48.43604651
      | -47.33522727
      | -46.28333333
      | -45.27717391
      | -44.31382979
      | -43.390625
      | -42.50510204
      | -41.655
      | 0
      | 41.655
      | 42.50510204
      | 43.390625
      | 44.31382979
      | 45.27717391
      | 46.28333333
      | 47.33522727
      | 48.43604651
      | 49.58928571
      | 50.79878049
      | 52.06875
      | 53.40384615
      | 54.80921053
      | 56.29054054
      | 57.85416667
      | 59.50714286
      | 61.25735294
      | 63.11363636
      | 65.0859375
      | 67.18548387
      | 69.425
      | 71.81896552
      | 74.38392857
      | 77.13888889
      | 80.10576923
      | 83.31
      | ]
      | [-56.56514507
      | -53.54549481
      | -50.84271532
      | -48.40677775
      | -46.19848973
      | -44.1864403
      | -42.34501024
      | -40.65301137
      | -39.09271935
      | -37.64916478
      | -36.30960068
      | -35.06309421
      | -33.9002085
      | -32.81275112
      | -31.7935729
      | -30.83640531
      | -29.93572777
      | -29.08665866
      | -28.28486498
      | -27.52648702
      | -26.80807528
      | -26.1265372
      | -25.47909206
      | -24.86323253
      | -24.27669186
      | -23.71741561
      | 0
      | 19.43364926
      | 19.81507719
      | 20.21246499
      | 20.62689117
      | 21.05953958
      | 21.51171342
      | 21.98485165
      | 22.48054833
      | 23.00057556
      | 23.54691095
      | 24.12177053
      | 24.72764882
      | 25.36736764
      | 26.04413644
      | 26.76162747
      | 27.52407048
      | 28.33637359
      | 29.20427963
      | 30.13457154
      | 31.13534711
      | 32.21639355
      | 33.38971041
      | 34.67025898
      | 36.07707064
      | 37.63494871
      | 39.37720355
      | ]
  steering wheel angle (pinion) to rack dispacement : Lookup_n-D  NumberOfTableDimensions=1  BreakpointsForDimension1=|  Table=|  RndMeth=Simplest  InputSameDT=on
      BreakpointsForDimension1=|
      | [-807.1596203
      | -767.526082
      | -732.1745847
      | -700.3549602
      | -671.5005069
      | -645.1711331
      | -621.017417
      | -598.7568399
      | -578.1574816
      | -559.0264878
      | -541.2017003
      | -524.5454483
      | -508.9398532
      | -494.2832202
      | -480.4872231
      | -467.4746805
      | -455.1777777
      | -443.5366317
      | -432.4981203
      | -422.0149202
      | -412.0447096
      | -402.5495034
      | -393.495094
      | -384.8505798
      | -376.5879637
      | -368.6818104
      | 0
      | 368.6818104
      | 376.5879637
      | 384.8505798
      | 393.495094
      | 402.5495034
      | 412.0447096
      | 422.0149202
      | 432.4981203
      | 443.5366317
      | 455.1777777
      | 467.4746805
      | 480.4872231
      | 494.2832202
      | 508.9398532
      | 524.5454483
      | 541.2017003
      | 559.0264878
      | 578.1574816
      | 598.7568399
      | 621.017417
      | 645.1711331
      | 671.5005069
      | 700.3549602
      | 732.1745847
      | 767.526082
      | 807.1596203
      | ]
      Table=|
      | [-83.31
      | -80.10576923
      | -77.13888889
      | -74.38392857
      | -71.81896552
      | -69.425
      | -67.18548387
      | -65.0859375
      | -63.11363636
      | -61.25735294
      | -59.50714286
      | -57.85416667
      | -56.29054054
      | -54.80921053
      | -53.40384615
      | -52.06875
      | -50.79878049
      | -49.58928571
      | -48.43604651
      | -47.33522727
      | -46.28333333
      | -45.27717391
      | -44.31382979
      | -43.390625
      | -42.50510204
      | -41.655
      | 0
      | 41.655
      | 42.50510204
      | 43.390625
      | 44.31382979
      | 45.27717391
      | 46.28333333
      | 47.33522727
      | 48.43604651
      | 49.58928571
      | 50.79878049
      | 52.06875
      | 53.40384615
      | 54.80921053
      | 56.29054054
      | 57.85416667
      | 59.50714286
      | 61.25735294
      | 63.11363636
      | 65.0859375
      | 67.18548387
      | 69.425
      | 71.81896552
      | 74.38392857
      | 77.13888889
      | 80.10576923
      | 83.31
      | ]
  Right wheel steer ground (deg) : Outport  VectorParamsAs1DForOutWhenUnconnected=off
  Left wheel steer ground (deg) : Outport  Port=2  VectorParamsAs1DForOutWhenUnconnected=off
  wires:
  steering wheel angle deg/1 -> Deadband Deg/1
  steering wheel angle (pinion) to rack dispacement/1 -> Left wheel rack displacement to ground steering angle1/1, Right wheel rack displacement to ground steering angle/1
  Right wheel rack displacement to ground steering angle/1 -> Gain/1
  Left wheel rack displacement to ground steering angle1/1 -> Gain1/1
  Gain/1 -> Right wheel steer ground (deg)/1
  Gain1/1 -> Left wheel steer ground (deg)/1
  Deadband Deg/1 -> steering wheel angle (pinion) to rack dispacement/1

== system V2X_UDP_SCLX_Control_2019b/Subsystem2/PSG_first/Body Fixed Vehicle Dynamics/8dof_vehicle ==
  Tdf : Inport
  Tbfl : Inport  Port=2
  Tbfr : Inport  Port=3
  Tbrl : Inport  Port=4
  Tbrr : Inport  Port=5
  In7 : Inport  Port=6
  Fax : Inport  Port=7
  Fr : Inport  Port=8
  slope : Inport  Port=9
  deltaFL : Inport  Port=10
  deltaRL : Inport  Port=11
  V_ini : Inport  Port=12
  yaw_ini : Inport  Port=13
  vy_ini : Inport  Port=14
  4tyre_torque : Subsystem
  Bus Selector1 : BusSelector  OutputSignals=Fx_FL,Fx_FR,Fx_RL,Fx_RR,Fy_FL,Fy_FR
  Bus Selector2 : BusSelector  OutputSignals=Fy_FL,Fy_FR,Fy_RL,Fy_RR,Fx_FL,Fx_FR
  Bus Selector3 : BusSelector  OutputSignals=Fx_FL,Fx_FR,Fx_RL,Fx_RR
  Bus Selector4 : BusSelector  OutputSignals=Fy_FL,Fy_FR,Fy_RL,Fy_RR,Fx_FL,Fx_FR,Fx_RL,Fx_RR
  Constant1 : Constant  Value=0
  Gain2 : Gain  Gain=-1
  "Pitch " : Subsystem
  Roll : Subsystem
  Switch{,1..3} (4 alike) : Switch
  Yaw Dynamics : Subsystem
  deltaFL1 : InportShadow  Port=10
  deltaFL2 : InportShadow  Port=10
  deltaRL1 : InportShadow  Port=11
  deltaRL2 : InportShadow  Port=11
  lateral : Subsystem
  longitudinal : Subsystem
  omegafl : Outport  VectorParamsAs1DForOutWhenUnconnected=off
  omegafr : Outport  Port=2  VectorParamsAs1DForOutWhenUnconnected=off
  omegarl : Outport  Port=3  VectorParamsAs1DForOutWhenUnconnected=off
  omegarr : Outport  Port=4  VectorParamsAs1DForOutWhenUnconnected=off
  ax : Outport  Port=5  VectorParamsAs1DForOutWhenUnconnected=off
  Vx : Outport  Port=6  VectorParamsAs1DForOutWhenUnconnected=off
  Yaw Rate : Outport  Port=7  VectorParamsAs1DForOutWhenUnconnected=off
  Yaw angle : Outport  Port=8  VectorParamsAs1DForOutWhenUnconnected=off
  ay : Outport  Port=9  VectorParamsAs1DForOutWhenUnconnected=off
  Vy : Outport  Port=10  VectorParamsAs1DForOutWhenUnconnected=off
  "Veh Sideslip, Beta" : Outport  Port=11  VectorParamsAs1DForOutWhenUnconnected=off
  Pitch : Outport  Port=12  VectorParamsAs1DForOutWhenUnconnected=off
  Pitch_rate : Outport  Port=13  VectorParamsAs1DForOutWhenUnconnected=off
  "Roll " : Outport  Port=14  VectorParamsAs1DForOutWhenUnconnected=off
  Roll Rate : Outport  Port=15  VectorParamsAs1DForOutWhenUnconnected=off
  wires:
  V_ini/1 -> longitudinal/21(V_ini), 4tyre_torque/10(V_ini)
  vy_ini/1 -> lateral/17(vy_ini)
  yaw_ini/1 -> Yaw Dynamics/17(yaw_ini)
  Fax/1 -> longitudinal/7(Fax)
  lateral/2(Vy1) -> Vy/1, longitudinal/10(Vy)
  In7/1 -> Bus Selector4/1, Bus Selector3/1, Bus Selector1/1, Bus Selector2/1
  Bus Selector1/2 -> longitudinal/2(In2)  "<Fx_FR>"
  Bus Selector1/1 -> longitudinal/1(In1)  "<Fx_FL>"
  Bus Selector1/3 -> longitudinal/3(In5)  "<Fx_RL>"
  Bus Selector1/4 -> longitudinal/4(In6)  "<Fx_RR>"
  Fr/1 -> longitudinal/8(Fr)
  slope/1 -> longitudinal/9(slope)
  lateral/1(ay1) -> ay/1
  deltaFL/1 -> longitudinal/11(deltaFL)
  Bus Selector1/5 -> longitudinal/5(In3)  "<Fy_FL>"
  Bus Selector1/6 -> longitudinal/6(In4)  "<Fy_FR>"
  longitudinal/2(Vx) -> Vx/1, Gain2/1, Yaw Dynamics/1(Vx), lateral/7(Vx1)
  lateral/3(Veh Sideslip angle,Beta1) -> "Veh Sideslip, Beta"/1, Yaw Dynamics/2(Beta)
  deltaFL2/1 -> lateral/8(deltaFL)
  Bus Selector2/4 -> lateral/4(In10)  "<Fy_RR>"
  Bus Selector2/5 -> lateral/5(In11)  "<Fx_FL>"
  Bus Selector2/3 -> lateral/3(In9)  "<Fy_RL>"
  Bus Selector2/2 -> lateral/2(In8)  "<Fy_FR>"
  Bus Selector2/6 -> lateral/6(In12)  "<Fx_FR>"
  Bus Selector2/1 -> lateral/1(In7)  "<Fy_FL>"
  longitudinal/1(ax) -> ax/1
  deltaRL/1 -> longitudinal/12(deltaFR)
  deltaRL2/1 -> lateral/9(deltaFR)
  Yaw Dynamics/2(Yaw Rate) -> Yaw Rate/1, Roll/3(yaw_rate), longitudinal/19(yaw_rate), lateral/15(yaw_rate), "Pitch "/3(yaw_rate)
  Yaw Dynamics/1(Yaw angle) -> Yaw angle/1
  Bus Selector4/1 -> Yaw Dynamics/3(In3)  "<Fy_FL>"
  Bus Selector4/2 -> Yaw Dynamics/4(In4)  "<Fy_FR>"
  Bus Selector4/3 -> Yaw Dynamics/5(In5)  "<Fy_RL>"
  Bus Selector4/4 -> Yaw Dynamics/6(In6)  "<Fy_RR>"
  Bus Selector4/5 -> Yaw Dynamics/7(In1)  "<Fx_FL>"
  Bus Selector4/6 -> Yaw Dynamics/8(In2)  "<Fx_FR>"
  Bus Selector4/7 -> Yaw Dynamics/9(In7)  "<Fx_RL>"
  Bus Selector4/8 -> Yaw Dynamics/10(In8)  "<Fx_RR>"
  deltaFL1/1 -> Yaw Dynamics/11(In10)
  deltaRL1/1 -> Yaw Dynamics/12(In11)
  longitudinal/3(Fx) -> Yaw Dynamics/13(Fx), "Pitch "/1(Fx)
  lateral/4(Fy) -> Roll/1(Fy), Yaw Dynamics/14(Fy)
  Roll/2(roll) -> longitudinal/16(roll), lateral/12(roll), "Pitch "/2(roll), Yaw Dynamics/15(roll), "Roll "/1
  Roll/1(roll_rate) -> Roll Rate/1, longitudinal/17(roll_rate), lateral/13(roll_rate), "Pitch "/4(roll_rate)
  "Pitch "/2(pitch) -> Pitch/1, longitudinal/13(pitch), lateral/10(pitch), Yaw Dynamics/16("pitch "), Roll/2(pitch)
  "Pitch "/1(pitch_rate) -> longitudinal/14(pitch_rate), lateral/11(pitch_rate), Roll/4(pitch_rate), Pitch_rate/1
  Roll/3(Roll Accel) -> longitudinal/18(roll_accel), lateral/14(roll_accel)
  Yaw Dynamics/3(Yaw Accel) -> longitudinal/20(yaw_accel), lateral/16(yaw_accel)
  "Pitch "/3(pitch Accel) -> longitudinal/15(pitch_accel)
  4tyre_torque/1(omega_fl) -> omegafl/1
  Tbrl/1 -> Switch/3
  4tyre_torque/2(omega_fr) -> omegafr/1
  4tyre_torque/3(omega_rl) -> omegarl/1
  4tyre_torque/4(omega_rr) -> omegarr/1
  Tdf/1 -> 4tyre_torque/1(Tdf)
  Gain2/1 -> Switch/2, Switch1/2, Switch2/2, Switch3/2
  Tbfl/1 -> Switch1/3
  Constant1/1 -> Switch1/1, Switch2/1, Switch/1, Switch3/1
  Tbfr/1 -> Switch2/3
  Tbrr/1 -> Switch3/3
  Switch3/1 -> 4tyre_torque/5(Tbrr)
  Switch2/1 -> 4tyre_torque/3(Tbfr)
  Bus Selector3/1 -> 4tyre_torque/6(Fxfl)  "<Fx_FL>"
  Bus Selector3/2 -> 4tyre_torque/7(Fxfr)  "<Fx_FR>"
  Bus Selector3/3 -> 4tyre_torque/8(Fxrl)  "<Fx_RL>"
  Bus Selector3/4 -> 4tyre_torque/9(Fxrr)  "<Fx_RR>"
  Switch1/1 -> 4tyre_torque/2(Tbfl)
  Switch/1 -> 4tyre_torque/4(Tbrl)

== system V2X_UDP_SCLX_Control_2019b/Subsystem2/PSG_first/Body Fixed Vehicle Dynamics/Brakes ==
  note: 0-100
  lambda : Inport
  brake postion : Inport  Port=2
  "-1 " : Gain  Commented=on  Gain=-1
  Bus Selector : BusSelector  OutputSignals=signal1,signal2,signal3,signal4
  Constant : Constant  Commented=on  Value=0
  Constant1 : Constant  Value=0
  Constant2 : Constant  Value=0
  Delay{,1..3} (4 alike) : Delay  DelayLength=6  InitialCondition=0
  From : From  Commented=on  GotoTag=Des_Torque
  Front Brake Torque vs Pressure : Gain  Gain=300
  Front Prop Valve : Gain
  Rear Brake Torque vs Pressure1 : Gain  Gain=150
  Rear Prop Valve : Lookup_n-D  NumberOfTableDimensions=1  BreakpointsForDimension1=[0 2.5 3.5]  Table=[0 2.5 2.8]  DiagnosticForOutOfRangeInput=Warning  RndMeth=Simplest  InputSameDT=on
  Switch : Switch  Commented=on
  Switch1 : Switch  Threshold=0.12
  Switch2 : Switch  Threshold=0.12
  Switch3 : Switch  Threshold=0.15
  Switch4 : Switch  Threshold=0.15
  Terminator : Terminator  Commented=on
  brake position to master cylinder pressure : Gain  Gain=.0345
  Tbfl : Outport  VectorParamsAs1DForOutWhenUnconnected=off
  Tbfr : Outport  Port=2  VectorParamsAs1DForOutWhenUnconnected=off
  Tbrl : Outport  Port=3  VectorParamsAs1DForOutWhenUnconnected=off
  Tbrr : Outport  Port=4  VectorParamsAs1DForOutWhenUnconnected=off
  wires:
  Delay3/1 -> Tbrr/1
  Delay2/1 -> Tbrl/1
  Delay1/1 -> Tbfr/1
  Delay/1 -> Tbfl/1
  lambda/1 -> Bus Selector/1
  Switch/1 -> Terminator/1
  brake postion/1 -> brake position to master cylinder pressure/1
  "-1 "/1 -> Switch/3
  From/1 -> Switch/2, "-1 "/1
  Constant/1 -> Switch/1
  brake position to master cylinder pressure/1 -> Front Prop Valve/1, Rear Prop Valve/1
  Front Prop Valve/1 -> Front Brake Torque vs Pressure/1
  Constant2/1 -> Switch3/1, Switch4/1
  Bus Selector/4 -> Switch4/2  "<signal4>"
  Bus Selector/3 -> Switch3/2  "<signal3>"
  Bus Selector/2 -> Switch2/2  "<signal2>"
  Front Brake Torque vs Pressure/1 -> Switch1/3, Switch2/3
  Constant1/1 -> Switch1/1, Switch2/1
  Bus Selector/1 -> Switch1/2  "<signal1>"
  Switch4/1 -> Delay3/1
  Switch3/1 -> Delay2/1
  Switch2/1 -> Delay1/1
  Switch1/1 -> Delay/1
  Rear Brake Torque vs Pressure1/1 -> Switch3/3, Switch4/3
  Rear Prop Valve/1 -> Rear Brake Torque vs Pressure1/1

== system V2X_UDP_SCLX_Control_2019b/Subsystem2/PSG_first/Body Fixed Vehicle Dynamics/Driving Resistance Subsystem ==
  Vx : Inport
  Aerodynamic Resistance : Subsystem
  Rolling resistance : Subsystem
  Fax : Outport  VectorParamsAs1DForOutWhenUnconnected=off
  Fr : Outport  Port=2  VectorParamsAs1DForOutWhenUnconnected=off
  wires:
  Vx/1 -> Aerodynamic Resistance/1(Vx), Rolling resistance/1(Vx)
  Aerodynamic Resistance/1(Fa) -> Fax/1
  Rolling resistance/1(Fr) -> Fr/1
